simulink model "proj_ish"  (R2023a)
settings: Solver=FixedStepAuto  StartTime=0.0  StopTime=1000  FixedStep=0.01  RelTol=1e-3
values from neighbouring files (symbols this model uses):
  barrier_dist01 = 1300    [main_proj.m]
  barrier_dist02 = barrier_dist01+barrier_dist12    (= 10600)    [main_proj.m]
  barrier_dist03 = barrier_dist02+barrier_dist23    (= 21900)    [main_proj.m]
  barrier_dist04 = barrier_dist03+barrier_dist34    (= 53200)    [main_proj.m]
  L = 62832    [main_proj.m]
  start_times = [0 50 240]    [main_proj.m]
  train_acc_close = (30-50)/25    (= -0.8)    [main_proj.m]
  train_acc_passed = (50-30)/2.5    (= 8)    [main_proj.m]
  train_velocity_far = 50    [main_proj.m]
  trains = 3    [main_proj.m]
  V = 28    [main_proj.m]
  v = 0.15*V    (= 4.2)    [main_proj.m]
undefined symbols (not defined in the file or in its folder): a_cruise, a_cruise_stop, a_stop_start, converter_data, downtab, downth, emap, Iei, nevec, thvec, uptab, upth, vehicledata
(part 1 of 2)
settings Model: NumberOfSteps=100  Creator=Alex  LastModifiedBy=Alex

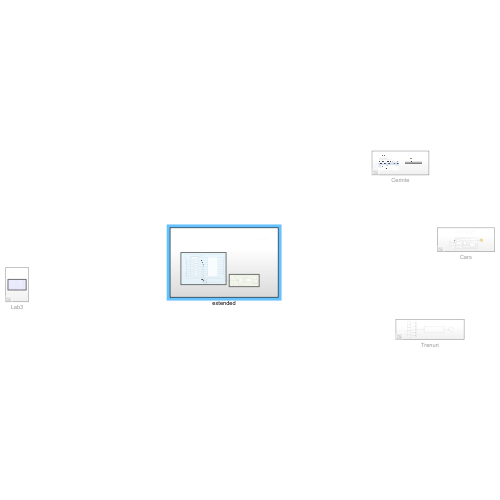
[thumbnail: Simulink's stored preview of the top-level diagram]
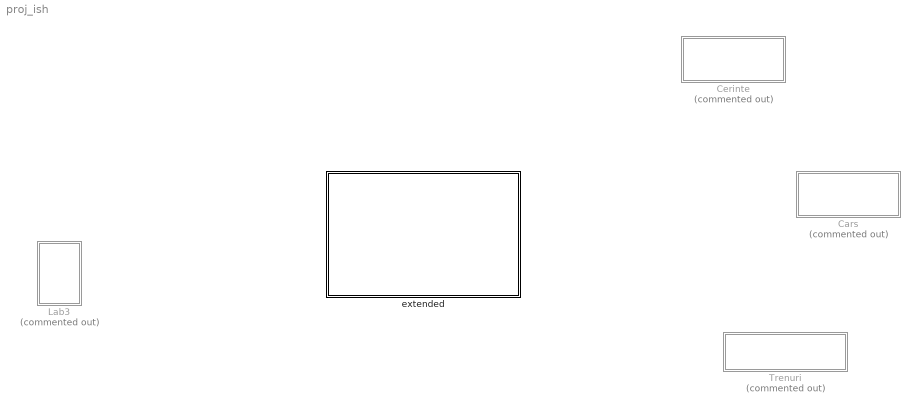
== system proj_ish ==
  Cars : Subsystem  Commented=on
  Cerinte : Subsystem  Commented=on
  Lab3 : Subsystem  Commented=on
  Trenuri : Subsystem  Commented=on
  extended : Subsystem

== system proj_ish/Cars ==
  Car : Subsystem  Commented=on
  Car Controller : Stateflow chart  Commented=on  TreatAsAtomicUnit=on
  Engine : Subsystem
  PlotResults : Scope  NumInputPorts=3
  Scope1 : Scope  Commented=on
  ShiftLogic : Stateflow chart  TreatAsAtomicUnit=on
  Step : Step  Time=50  Before=50  After=0  SampleTime=0
  Step1 : Step  Time=50  After=500  SampleTime=0
  Transmission : Subsystem
  Vehicle : Subsystem  mask(vehicle model){Rfd=vehicledata(1), rload0=vehicledata(2), rload2=vehicledata(3), Rw=vehicledata(4), Iv=vehicledata(5), N20=vehicledata(6)/vehicledata(4)*vehicledata(1)}
      mask prompts: Rfd "final drive ratio"; rload0 "drag friction at wheels"; rload2 "aerodynamic drag"; Rw "wheel radius"; Iv "vehicle inertia"; N20 "initial transmission output speed"
      mask help: vehicle dynamics: torque input from trans., outputs are input speed (transmission output) and vehicle speed
      mask Display: image('$imagefile') % use "Edit Image" on toolstrip to change.
  wires:
  Car/1(pozitie) -> Car Controller/1(pzoitie), Scope1/1
  Car Controller/1(stare_masina) -> Car/1(stare_masina)
  Transmission/2(Tout) -> Vehicle/1(OutputTorque)  "OutputTorque"
  Transmission/1(Ti) -> Engine/1(Ti)  "ImpellerTorque"
  ShiftLogic/1(Gear) -> Transmission/2(Gear)
  Engine/1(Ne) -> Transmission/1(Ne), PlotResults/2  "EngineRPM"
  Vehicle/1(VehicleSpeed) -> ShiftLogic/2(VehicleSpeed), PlotResults/3  "VehicleSpeed"
  Step1/1 -> Vehicle/2(BrakeTorque)  "Brake"
  Step/1 -> ShiftLogic/1(Throttle), Engine/2(Throttle), PlotResults/1  "Throttle"
  Vehicle/2(TransmissionRPM) -> Transmission/3(Nout)  "TransmissionRPM"

== system proj_ish/Cerinte ==
  note: trenul este in starea aproape, deci are viteza 30mps
      | evenimentul de "aproape" se genereaza la 1000m distanta de bariera
      | Durata propriu zisa de inchidere a barierei este 90/9=10 secunde
      | Trenul ajunge de la 1000m la 10m (pragul limita considerat) distanta de bariera in 990/30=33 secunde
      | Din cele 33 secunde, 10 se aloca pentru coborarea barierei
      | Deci intarzierea maxima pe care o poate avea controller-ul pentru a ne asigura ca bariera va fi complet inchisa la momentul in care trenul intra in intervalul +-10m este u=23 secunde
  note: r=10km => C=2*pi*r=62832m

== system proj_ish/Lab3 ==
  note: Lab 3
  Bariera : Subsystem  Commented=on
  Control bariera : Subsystem  Commented=on
  Controller : Stateflow chart  Commented=on  TreatAsAtomicUnit=on
  Scope : Scope  Commented=on  NumInputPorts=2
  Tren : Subsystem  Commented=on
  wires:
  Controller/1(starebariera) -> Bariera/1(stare_bariera)
  Bariera/1(y) -> Controller/1(y), Scope/2
  Controller/2(starectrl) -> Control bariera/1(stare_control)
  Control bariera/1(z) -> Controller/2(z)
  Tren/1(x) -> Controller/3(x), Scope/1
  Controller/3(staretren) -> Tren/1(stare_tren)

== system proj_ish/Trenuri ==
  Mux : Mux  Commented=on  Inputs=5
  Scope1 : Scope  Commented=on
  Step{,1..4} (5 alike) : Step  Commented=on  Time=0  SampleTime=0
  Trenuri : Subsystem  Commented=on
  wires:
  Step/1 -> Mux/1
  Mux/1 -> Trenuri/1(stari_trenuri)
  Step2/1 -> Mux/3
  Trenuri/1(x) -> Scope1/1
  Step3/1 -> Mux/4
  Step1/1 -> Mux/2
  Step4/1 -> Mux/5

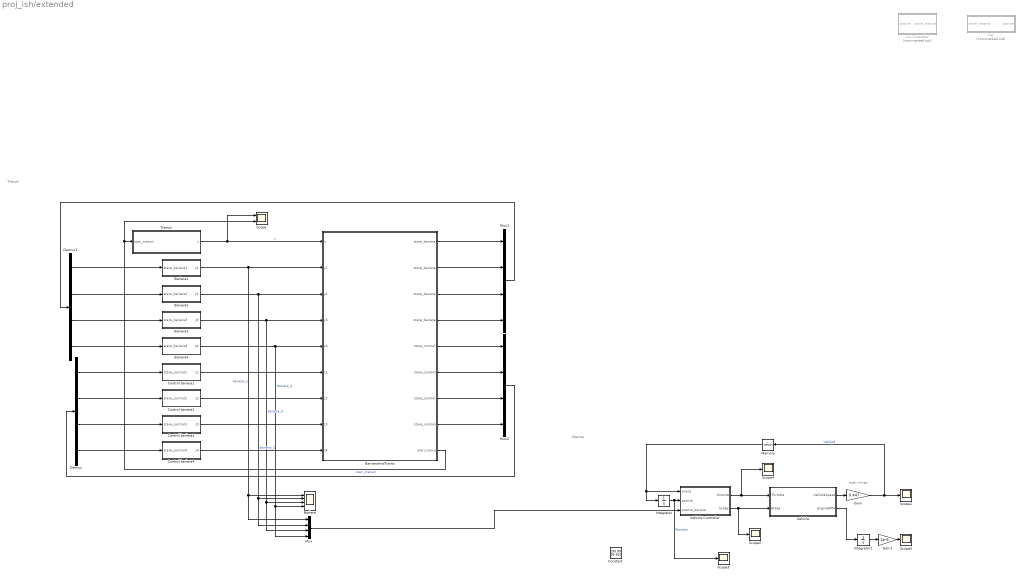
== system proj_ish/extended ==
  note: Masina
  note: Trenuri
  note: mph->mps
  Bariera1 : Subsystem
  Bariera2 : Subsystem
  Bariera3 : Subsystem
  Bariera4 : Subsystem
  Bariere : Scope  NumInputPorts=4
  BarriersAndTrains : Stateflow chart  TreatAsAtomicUnit=on
  Car : Subsystem  Commented=on
  Car Controller : Stateflow chart  Commented=on  TreatAsAtomicUnit=on
  Constant : Constant  Value=[90 90 90 90]
  Control bariera1 : Subsystem
  Control bariera2 : Subsystem
  Control bariera3 : Subsystem
  Control bariera4 : Subsystem
  Demux : Demux
  Demux1 : Demux
  Gain : Gain  Gain=0.447
  Gain1 : Gain  Gain=2e-6
  Integrator : Integrator
  Integrator1 : Integrator
  Memory : Memory
  Mux : Mux
  Mux1 : Mux
  Mux2 : Mux
  Scope : Scope  NumInputPorts=2
  Scope{1..5} (5 alike) : Scope
  Trenuri : Subsystem
  Vehicle : Subsystem
  Vehicle Controller : Stateflow chart  TreatAsAtomicUnit=on
      settings: PortSchema="{\"entries\":[{\"content\":{\"sides\":[{\"content\":{\"connectorIds\":[\"In2\",\"In1\",\"In3\"]},\"type\":\"ConnectorPlacement.EquallySpacedRectSide\",\"uuid\":\"df773432-b911-4b0c-bdef-38af23bc8129\"},{\"content\":{\"connectorIds\":[\"Out1\",\"Out2\"],\"side\":\"RIGHT\"},\"type\":\"ConnectorPlacement.EquallySpacedRectSide\",\"uuid\":\"5ca2d89f-a3cb-4395-9b83-e502d168ef7e\"},{\"content\":{\"side\":\"TOP\"},\"type\":\"ConnectorPlacement.EquallySpacedRectSide\",\"uuid\":\"7df5f796-226c-4e0d-a429-f20110d7350f\"}]},\"type\":\"ConnectorPlacement.EquallySpacedConnector\",\"uuid\":\"5b5bbf8d-caf4-492a-a09a-43efcf324f87\"}],\"packageUris\":[\"http://schema.mathworks.com/mf0/Connector/R2020b\"],\"version\":\"1.0\"}"
  wires:
  Trenuri/1(x) -> Scope/1, BarriersAndTrains/1(x)  "x"
  Bariera1/1(y1) -> Mux/1, Bariere/1, BarriersAndTrains/2(y1)  "bariera_1"
  Bariera2/1(y2) -> Mux/2, Bariere/2, BarriersAndTrains/3(y2)  "bariera_2"
  Bariera3/1(y3) -> Mux/3, Bariere/3, BarriersAndTrains/4(y3)  "bariera_3"
  Bariera4/1(y4) -> BarriersAndTrains/5(y4), Mux/4, Bariere/4  "bariera_4"
  Control bariera3/1(z3) -> BarriersAndTrains/8(z3)
  Control bariera2/1(z2) -> BarriersAndTrains/7(z2)
  Control bariera1/1(z1) -> BarriersAndTrains/6(z1)
  Control bariera4/1(z4) -> BarriersAndTrains/9(z4)
  BarriersAndTrains/2(stare_bariera2) -> Mux1/2
  BarriersAndTrains/1(stare_bariera1) -> Mux1/1
  BarriersAndTrains/3(stare_bariera3) -> Mux1/3
  BarriersAndTrains/4(stare_bariera4) -> Mux1/4
  BarriersAndTrains/5(stare_control1) -> Mux2/1
  BarriersAndTrains/6(stare_control2) -> Mux2/2
  BarriersAndTrains/7(stare_control3) -> Mux2/3
  BarriersAndTrains/8(stare_control4) -> Mux2/4
  Mux2/1 -> Demux/1
  Demux/3 -> Control bariera3/1(stare_control3)
  Demux/2 -> Control bariera2/1(stare_control2)
  Demux/4 -> Control bariera4/1(stare_control4)
  Demux/1 -> Control bariera1/1(stare_control1)
  Demux1/1 -> Bariera1/1(stare_bariera1)
  Demux1/2 -> Bariera2/1(stare_bariera2)
  Demux1/3 -> Bariera3/1(stare_bariera3)
  Demux1/4 -> Bariera4/1(stare_bariera4)
  Mux1/1 -> Demux1/1
  BarriersAndTrains/9(stari_trenuri) -> Scope/2, Trenuri/1(stari_trenuri)  "stari_trenuri"
  Vehicle Controller/2(brake) -> Scope2/1, Vehicle/2(Brake)
  Integrator/1 -> Scope3/1, Vehicle Controller/1(pozitie)  "Position"
  Gain/1 -> Memory/1, Scope1/1  "VehSpd"
  Vehicle Controller/1(throttle) -> Scope4/1, Vehicle/1(Throttle)
  Memory/1 -> Integrator/1, Vehicle Controller/2(viteza)
  Vehicle/1(VehicleSpeed) -> Gain/1
  Mux/1 -> Vehicle Controller/3(pozitie_bariere)
  Vehicle/2(EngineRPM) -> Integrator1/1
  Integrator1/1 -> Gain1/1
  Gain1/1 -> Scope5/1

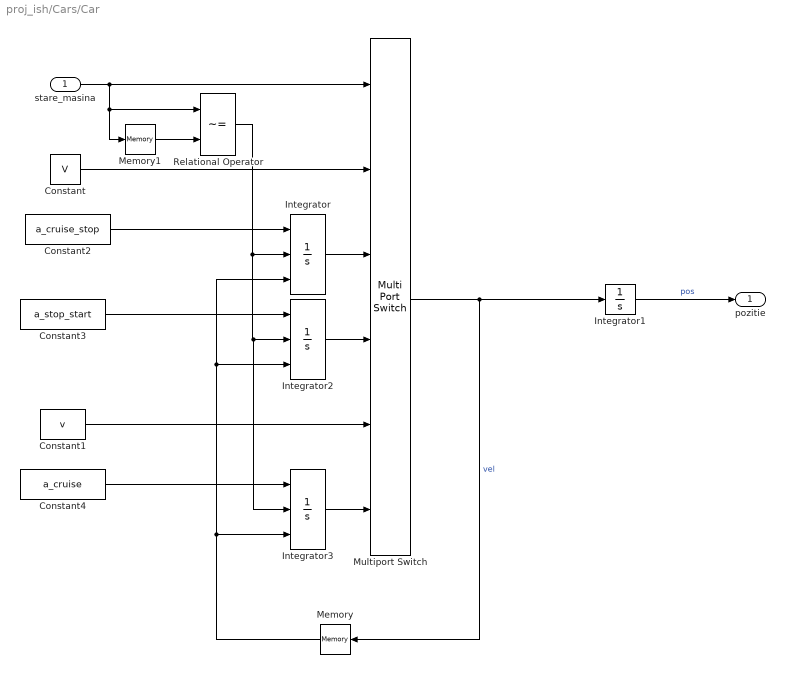
== system proj_ish/Cars/Car ==
  stare_masina : Inport
  Constant : Constant  Value=V
  Constant1 : Constant  Value=v
  Constant2 : Constant  Value=a_cruise_stop
  Constant3 : Constant  Value=a_stop_start
  Constant4 : Constant  Value=a_cruise
  Integrator : Integrator  ExternalReset=rising  InitialConditionSource=external  LimitOutput=on  UpperSaturationLimit=200  LowerSaturationLimit=0
  Integrator1 : Integrator
  Integrator2 : Integrator  ExternalReset=rising  InitialConditionSource=external  LimitOutput=on  UpperSaturationLimit=v  LowerSaturationLimit=0
  Integrator3 : Integrator  ExternalReset=rising  InitialConditionSource=external  LimitOutput=on  UpperSaturationLimit=V  LowerSaturationLimit=0
  Memory : Memory  InitialCondition=V
  Memory1 : Memory  InitialCondition=1
  Multiport Switch : MultiPortSwitch  Inputs=5  SaturateOnIntegerOverflow=off  InputSameDT=off
  Relational Operator : RelationalOperator  Operator=~=  OutDataTypeStr=boolean  RndMeth=Simplest  InputSameDT=off
  pozitie : Outport
  wires:
  Multiport Switch/1 -> Memory/1, Integrator1/1  "vel"
  stare_masina/1 -> Multiport Switch/1, Memory1/1, Relational Operator/1
  Integrator1/1 -> pozitie/1  "pos"
  Constant/1 -> Multiport Switch/2
  Integrator/1 -> Multiport Switch/3
  Integrator2/1 -> Multiport Switch/4
  Constant1/1 -> Multiport Switch/5
  Integrator3/1 -> Multiport Switch/6
  Memory/1 -> Integrator3/3, Integrator2/3, Integrator/3
  Memory1/1 -> Relational Operator/2
  Relational Operator/1 -> Integrator3/2, Integrator2/2, Integrator/2
  Constant2/1 -> Integrator/1
  Constant3/1 -> Integrator2/1
  Constant4/1 -> Integrator3/1

== system proj_ish/Cars/Engine ==
  note: Engine
  Ti : Inport  Unit=ft*lbf@torque
  Throttle : Inport  Port=2  Unit=%
  EnginePlusImpellerInertia : Gain  Gain=1/Iei  SaturateOnIntegerOverflow=on  OutDataTypeStr=Inherit: Same as input  ParamDataTypeStr=Inherit: Same as input
  EngineTorque : Lookup_n-D  BreakpointsForDimension1=thvec  BreakpointsForDimension2=nevec  Table=emap
      settings: InputPortMap=u0,u1
  Integrator : Integrator  InitialCondition=1000  LimitOutput=on  UpperSaturationLimit=6000  LowerSaturationLimit=600  ZeroCross=off
  Sum : Sum  Inputs=-+  InputSameDT=on  SaturateOnIntegerOverflow=on  OutDataTypeStr=Inherit: Same as first input
  Ne : Outport  Unit=rpm  VectorParamsAs1DForOutWhenUnconnected=off
  wires:
  Ti/1 -> Sum/1
  Throttle/1 -> EngineTorque/1
  Integrator/1 -> EngineTorque/2, Ne/1
  Sum/1 -> EnginePlusImpellerInertia/1
  EnginePlusImpellerInertia/1 -> Integrator/1
  EngineTorque/1 -> Sum/2

== system proj_ish/Cars/ShiftLogic/ComputeThreshold ==
  note: Threshold Calculation
  Gear : Inport
  Throttle : Inport  Port=2
  f : TriggerPort  TriggerType=function-call  VariantControl=(inherit)
      settings: CopyFcn=Stateflow.SLINSF.SimulinkMan.removeBlockPreDeleteFcn  PreDeleteFcn=Stateflow.SLINSF.SimulinkMan.unsafePredeleteFcn
  InterpDown : Lookup_n-D  BreakpointsForDimension1=downth  BreakpointsForDimension2=[1:4]  Table=downtab  OutDataTypeStr=double  InputSameDT=off  LockScale=on
      settings: InputPortMap=u0,u1
  InterpUp : Lookup_n-D  BreakpointsForDimension1=upth  BreakpointsForDimension2=[1:4]  Table=uptab  OutDataTypeStr=double  InputSameDT=off  LockScale=on
      settings: InputPortMap=u0,u1
  down_th : Outport  InitialOutput=0  VectorParamsAs1DForOutWhenUnconnected=off
  up_th : Outport  Port=2  InitialOutput=0  VectorParamsAs1DForOutWhenUnconnected=off
  wires:
  InterpUp/1 -> up_th/1
  InterpDown/1 -> down_th/1
  Throttle/1 -> InterpDown/1, InterpUp/1
  Gear/1 -> InterpDown/2, InterpUp/2

== system proj_ish/Cars/Transmission ==
  note: Transmission
  Ne : Inport  Unit=rpm
  Gear : Inport  Port=2  Unit=1
  Nout : Inport  Port=3  Unit=rpm
  TorqueConverter : Subsystem  mask(torque converter){speedratio=converter_data(:,1), Kfactor=converter_data(:,2), Torkratio=converter_data(:,3)}
      mask prompts: speedratio "speed ratio"; Kfactor "K factor"; Torkratio "torque ratio"
      mask help: torque converter
      mask Help: Torque converter input and output torques are computed as a function of the input and output speeds
      mask Display: plot([cos([90:10:450]*pi/180),.63*cos([90:10:450]*pi/180),.63*cos([90:10:240]*pi/180),cos([240:10:300]*pi/180),.63*cos([300]*pi/180)],[sin([90:10:450]*pi/180),.63*sin([90:10:450]*pi/180)+.1,.63*sin([90:10:240]*pi/180)+.1,sin([240:10:300]*pi/180),.63*sin([300]*pi/180)+.1])
  TransmissionRatio : Subsystem
  Ti : Outport  Unit=ft*lbf@torque  VectorParamsAs1DForOutWhenUnconnected=off
  Tout : Outport  Port=2  Unit=ft*lbf@torque  VectorParamsAs1DForOutWhenUnconnected=off
  wires:
  TransmissionRatio/1(Tout) -> Tout/1
  TorqueConverter/1(Ti) -> Ti/1
  Nout/1 -> TransmissionRatio/3(Nout)
  Gear/1 -> TransmissionRatio/2(Gear)
  Ne/1 -> TorqueConverter/1(Ne)
  TransmissionRatio/2(Nin) -> TorqueConverter/2(Nin)
  TorqueConverter/2(Tt) -> TransmissionRatio/1(Tin)  "TurbineTorque"

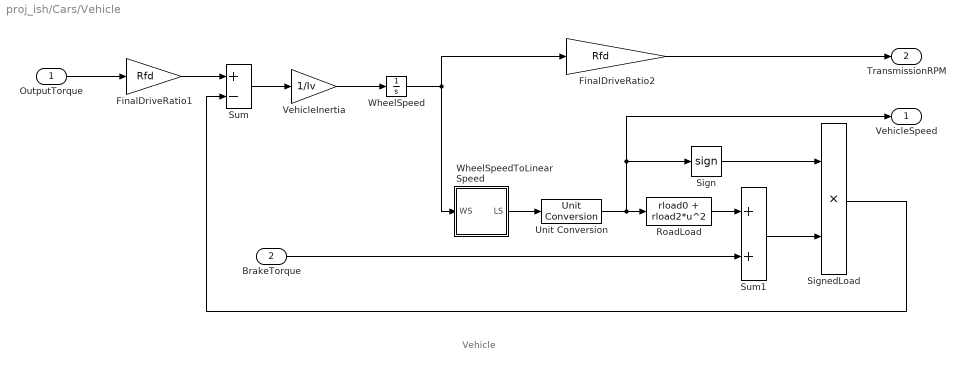
== system proj_ish/Cars/Vehicle ==
  note: Vehicle
  OutputTorque : Inport  Unit=ft*lbf@torque
  BrakeTorque : Inport  Port=2  Unit=ft*lbf@torque
  FinalDriveRatio1 : Gain  Gain=Rfd  SaturateOnIntegerOverflow=on  OutDataTypeStr=Inherit: Same as input  ParamDataTypeStr=Inherit: Same as input
  FinalDriveRatio2 : Gain  Gain=Rfd  SaturateOnIntegerOverflow=on  OutDataTypeStr=Inherit: Same as input  ParamDataTypeStr=Inherit: Same as input
  RoadLoad : Fcn  Expr=rload0 + rload2*u^2
  Sign : Signum
  SignedLoad : Product  InputSameDT=on  SaturateOnIntegerOverflow=on  OutDataTypeStr=Inherit: Same as first input
  Sum : Sum  Inputs=+-  InputSameDT=on  SaturateOnIntegerOverflow=on  OutDataTypeStr=Inherit: Same as first input
  Sum1 : Sum  InputSameDT=on  SaturateOnIntegerOverflow=on  OutDataTypeStr=Inherit: Same as first input
  Unit Conversion : UnitConversion
  VehicleInertia : Gain  Gain=1/Iv  SaturateOnIntegerOverflow=on  OutDataTypeStr=Inherit: Same as input  ParamDataTypeStr=Inherit: Same as input
  WheelSpeed : Integrator  InitialCondition=N20/Rfd  ZeroCross=off
  WheelSpeedToLinearSpeed : Subsystem
  VehicleSpeed : Outport  Unit=mph  VectorParamsAs1DForOutWhenUnconnected=off
  TransmissionRPM : Outport  Port=2  Unit=rpm  VectorParamsAs1DForOutWhenUnconnected=off
  wires:
  FinalDriveRatio2/1 -> TransmissionRPM/1
  BrakeTorque/1 -> Sum1/2
  Sum1/1 -> SignedLoad/2
  RoadLoad/1 -> Sum1/1
  Sign/1 -> SignedLoad/1
  SignedLoad/1 -> Sum/2
  OutputTorque/1 -> FinalDriveRatio1/1
  VehicleInertia/1 -> WheelSpeed/1
  Sum/1 -> VehicleInertia/1
  Unit Conversion/1 -> VehicleSpeed/1, Sign/1, RoadLoad/1
  WheelSpeed/1 -> WheelSpeedToLinearSpeed/1(WS), FinalDriveRatio2/1
  FinalDriveRatio1/1 -> Sum/1
  WheelSpeedToLinearSpeed/1(LS) -> Unit Conversion/1

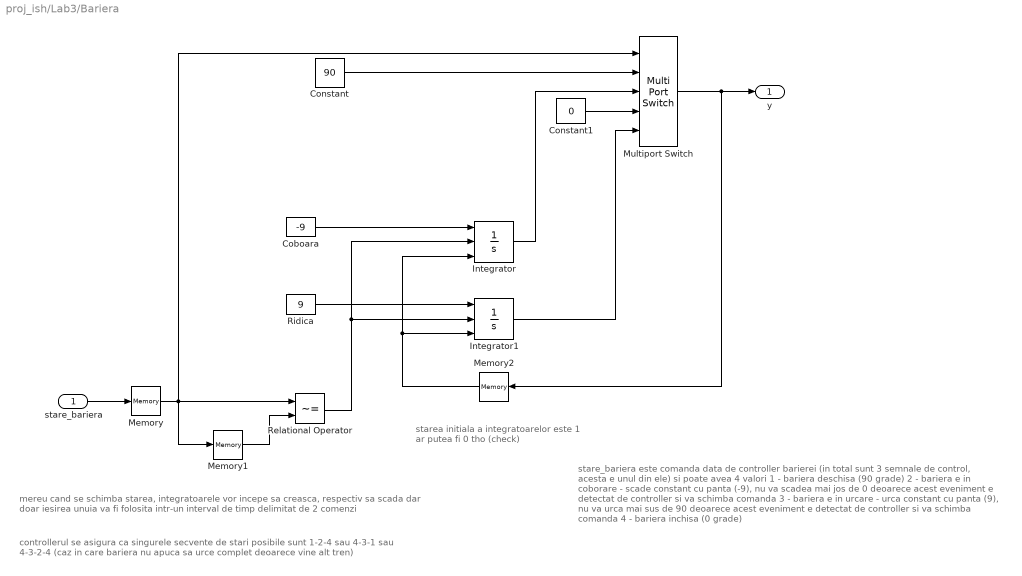
== system proj_ish/Lab3/Bariera ==
  note: controllerul se asigura ca singurele secvente de stari posibile sunt
      | 1-2-4
      | sau
      | 4-3-1
      | sau 4-3-2-4 (caz in care bariera nu apuca sa urce complet deoarece vine alt tren)
  note: mereu cand se schimba starea, integratoarele vor incepe sa creasca, respectiv sa scada
      | dar doar iesirea unuia va fi folosita intr-un interval de timp delimitat de 2 comenzi
  note: starea initiala a integratoarelor este 1
      | ar putea fi 0 tho (check)
  note: stare_bariera este comanda data de controller barierei (in total sunt 3 semnale de control, acesta e unul din ele) si poate avea 4 valori
      | 1 - bariera deschisa (90 grade)
      | 2 - bariera e in coborare - scade constant cu panta (-9), nu va scadea mai jos de 0 deoarece acest eveniment e detectat de controller si va schimba comanda
      | 3 - bariera e in urcare - urca constant cu panta (9), nu va urca mai sus de 90 deoarece acest eveniment e detectat de controller si va schimba comanda
      | 4 - bariera inchisa (0 grade)
  stare_bariera : Inport
  Coboara : Constant  Value=-9
  Constant : Constant  Value=90
  Constant1 : Constant  Value=0
  Integrator : Integrator  ExternalReset=rising  InitialConditionSource=external
  Integrator1 : Integrator  ExternalReset=rising  InitialConditionSource=external
  Memory : Memory  InitialCondition=1
  Memory1 : Memory  InitialCondition=1
  Memory2 : Memory
  Multiport Switch : MultiPortSwitch  Inputs=4  SaturateOnIntegerOverflow=off  InputSameDT=off
  Relational Operator : RelationalOperator  Operator=~=  OutDataTypeStr=boolean  RndMeth=Simplest  InputSameDT=off
  Ridica : Constant  Value=9
  y : Outport
  wires:
  Multiport Switch/1 -> Memory2/1, y/1
  Constant/1 -> Multiport Switch/2
  Coboara/1 -> Integrator/1
  Ridica/1 -> Integrator1/1
  Integrator/1 -> Multiport Switch/3
  stare_bariera/1 -> Memory/1
  Memory/1 -> Multiport Switch/1, Memory1/1, Relational Operator/1
  Memory1/1 -> Relational Operator/2
  Relational Operator/1 -> Integrator1/2, Integrator/2
  Integrator1/1 -> Multiport Switch/5
  Constant1/1 -> Multiport Switch/4
  Memory2/1 -> Integrator/3, Integrator1/3

== system proj_ish/Lab3/Control bariera ==
  note: iesirea z masoara cat timp a trecut de la ultima comanda de tip ridicare sau coborare
      | (scopul este modelarea unui delay intre momentul in care se ia decizia si momentul in care bariera executa comanda, modelarea propriu zisa se face in controller)
      |
      | daca controllerul e in starea de asteptare, atunci z=0
      | daca controllerul hotaraste comanda de ridicare sau coborare, se porneste un timer care se opreste cand are loc una din tranzitiile {3->1} {2->1} {3->2}
  note: stare_control este starea decizionala in care se afla controllerul
      | 1 - asteptare
      | 2 - comanda coborare
      | 3 - comanda ridicare
  stare_control : Inport
  Constant : Constant  Value=0
  Constant1 : Constant
  Constant2 : Constant
  Integrator : Integrator  ExternalReset=rising
  Memory : Memory  InitialCondition=1
  Memory1 : Memory  InitialCondition=1
  Multiport Switch : MultiPortSwitch  DataPortOrder=Specify indices  Inputs=2  DataPortIndices={0,1}  SaturateOnIntegerOverflow=off  InputSameDT=off
  Relational Operator : RelationalOperator  Operator=~=  OutDataTypeStr=boolean  RndMeth=Simplest  InputSameDT=off
  Relational Operator1 : RelationalOperator  Operator===  OutDataTypeStr=boolean  RndMeth=Simplest  InputSameDT=off
  z : Outport
  wires:
  Multiport Switch/1 -> z/1
  Constant/1 -> Multiport Switch/3
  stare_control/1 -> Relational Operator/1, Memory/1
  Memory/1 -> Relational Operator/2, Relational Operator1/1
  Constant1/1 -> Integrator/1
  Relational Operator/1 -> Integrator/2
  Integrator/1 -> Memory1/1
  Memory1/1 -> Multiport Switch/2
  Constant2/1 -> Relational Operator1/2
  Relational Operator1/1 -> Multiport Switch/1

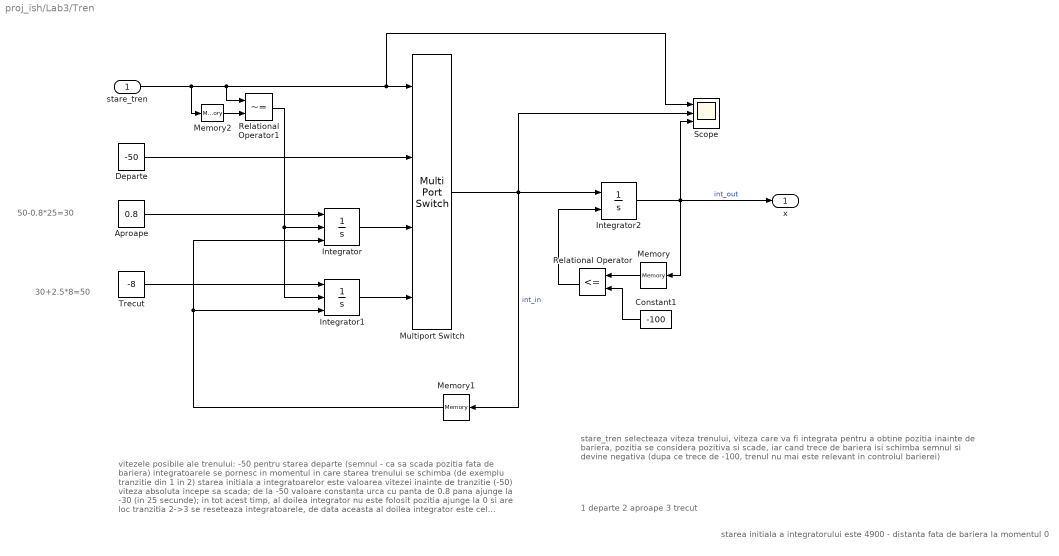
== system proj_ish/Lab3/Tren ==
  note: 30+2.5*8=50
  note: starea initiala a integratorului este 4900 - distanta fata de bariera la momentul 0
  note: 1 departe
      | 2 aproape
      | 3 trecut
  note: vitezele posibile ale trenului:
      | -50 pentru starea departe (semnul - ca sa scada pozitia fata de bariera)
      |
      | integratoarele se pornesc in momentul in care starea trenului se schimba (de exemplu tranzitie din 1 in 2)
      |
      | starea initiala a integratoarelor este valoarea vitezei inainte de tranzitie (-50)
      | viteza absoluta incepe sa scada; de la -50 valoare constanta urca cu panta de 0.8 pana ajunge la -30 (in 25 secunde); in tot acest timp, al doilea integrator nu este folosit
      |
      | pozitia ajunge la 0 si are loc tranzitia 2->3
      |
      | se reseteaza integratoarele, de data aceasta al doilea integrator este cel folosit; el are starea initiala -30 si scade cu o panta de -8
  note: 50-0.8*25=30
  note: stare_tren selecteaza viteza trenului, viteza care va fi integrata pentru a obtine pozitia
      | inainte de bariera, pozitia se considera pozitiva si scade, iar cand trece de bariera isi schimba semnul si devine negativa (dupa ce trece de -100, trenul nu mai este relevant in controlul barierei)
  stare_tren : Inport
  Aproape : Constant  Value=0.8
  Constant1 : Constant  Value=-100
  Departe : Constant  Value=-50
  Integrator : Integrator  ExternalReset=rising  InitialConditionSource=external
  Integrator1 : Integrator  ExternalReset=rising  InitialConditionSource=external
  Integrator2 : Integrator  ExternalReset=rising  InitialCondition=4900
  Memory : Memory
  Memory1 : Memory
  Memory2 : Memory  InitialCondition=1
  Multiport Switch : MultiPortSwitch  SaturateOnIntegerOverflow=off  InputSameDT=off
  Relational Operator : RelationalOperator  Operator=<=  OutDataTypeStr=boolean  RndMeth=Simplest  InputSameDT=off
  Relational Operator1 : RelationalOperator  Operator=~=  OutDataTypeStr=boolean  RndMeth=Simplest  InputSameDT=off
  Scope : Scope  NumInputPorts=3
  Trecut : Constant  Value=-8
  x : Outport
  wires:
  Departe/1 -> Multiport Switch/2
  stare_tren/1 -> Memory2/1, Scope/1, Multiport Switch/1, Relational Operator1/1
  Aproape/1 -> Integrator/1
  Trecut/1 -> Integrator1/1
  Integrator2/1 -> Scope/3, x/1, Memory/1  "int_out"
  Constant1/1 -> Relational Operator/2
  Memory/1 -> Relational Operator/1
  Relational Operator/1 -> Integrator2/2
  Multiport Switch/1 -> Scope/2, Memory1/1, Integrator2/1  "int_in"
  Integrator/1 -> Multiport Switch/3
  Integrator1/1 -> Multiport Switch/4
  Memory1/1 -> Integrator/3, Integrator1/3
  Memory2/1 -> Relational Operator1/2
  Relational Operator1/1 -> Integrator/2, Integrator1/2

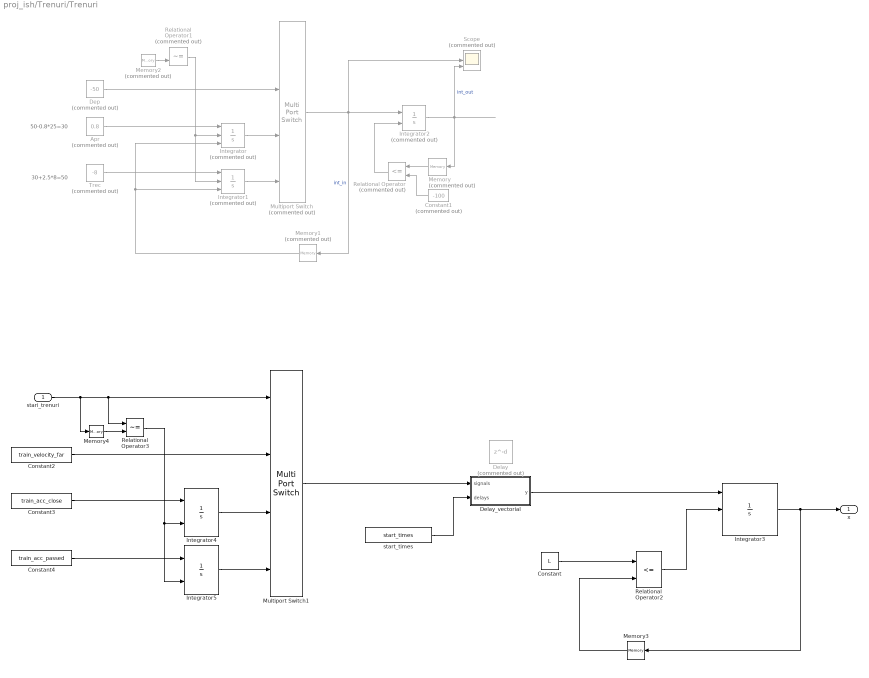
== system proj_ish/Trenuri/Trenuri ==
  note: 30+2.5*8=50
  note: 50-0.8*25=30
  stari_trenuri : Inport
  Apr : Constant  Commented=on  Value=0.8
  Constant : Constant  Value=L
  Constant1 : Constant  Commented=on  Value=-100
  Constant2 : Constant  Value=train_velocity_far
  Constant3 : Constant  Value=train_acc_close
  Constant4 : Constant  Value=train_acc_passed
  Delay : Delay  Commented=on  DelayLengthSource=Input port
      settings: InputPortMap=u0,p1
  Delay_vectorial : MATLAB Function  TreatAsAtomicUnit=on
  Dep : Constant  Commented=on  Value=-50
  Integrator : Integrator  Commented=on  ExternalReset=rising  InitialConditionSource=external
  Integrator1 : Integrator  Commented=on  ExternalReset=rising  InitialConditionSource=external
  Integrator2 : Integrator  Commented=on  ExternalReset=rising  InitialCondition=4900
  Integrator3 : Integrator  ExternalReset=rising  InitialConditionSource=external
  Integrator4 : Integrator  ExternalReset=rising
  Integrator5 : Integrator  ExternalReset=rising
  Memory : Memory  Commented=on
  Memory1 : Memory  Commented=on
  Memory2 : Memory  Commented=on  InitialCondition=1
  Memory3 : Memory
  Memory4 : Memory  InitialCondition=ones(1,trains)
  Multiport Switch : MultiPortSwitch  Commented=on  SaturateOnIntegerOverflow=off  InputSameDT=off
  Multiport Switch1 : MultiPortSwitch  SaturateOnIntegerOverflow=off  InputSameDT=off
  Relational Operator : RelationalOperator  Commented=on  Operator=<=  OutDataTypeStr=boolean  RndMeth=Simplest  InputSameDT=off
  Relational Operator1 : RelationalOperator  Commented=on  Operator=~=  OutDataTypeStr=boolean  RndMeth=Simplest  InputSameDT=off
  Relational Operator2 : RelationalOperator  Operator=<=  OutDataTypeStr=boolean  RndMeth=Simplest  InputSameDT=off
  Relational Operator3 : RelationalOperator  Operator=~=  OutDataTypeStr=boolean  RndMeth=Simplest  InputSameDT=off
  Scope : Scope  Commented=on  NumInputPorts=3
  Trec : Constant  Commented=on  Value=-8
  start_times : Constant  Value=start_times
  x : Outport
  wires:
  Dep/1 -> Multiport Switch/2
  ? -> Memory2/1, Scope/1, Multiport Switch/1, Relational Operator1/1
  Apr/1 -> Integrator/1
  Trec/1 -> Integrator1/1
  Integrator2/1 -> Scope/3, Memory/1  "int_out"
  Constant1/1 -> Relational Operator/2
  Memory/1 -> Relational Operator/1
  Relational Operator/1 -> Integrator2/2
  Multiport Switch/1 -> Scope/2, Memory1/1, Integrator2/1  "int_in"
  Integrator/1 -> Multiport Switch/3
  Integrator1/1 -> Multiport Switch/4
  Memory1/1 -> Integrator/3, Integrator1/3
  Memory2/1 -> Relational Operator1/2
  Relational Operator1/1 -> Integrator/2, Integrator1/2
  Multiport Switch1/1 -> Delay_vectorial/1(signals)
  stari_trenuri/1 -> Multiport Switch1/1, Relational Operator3/1, Memory4/1
  Integrator3/1 -> Memory3/1, x/1
  Constant2/1 -> Multiport Switch1/2
  start_times/1 -> Delay_vectorial/2(delays)
  Integrator4/1 -> Multiport Switch1/3
  Integrator5/1 -> Multiport Switch1/4
  Delay_vectorial/1(y) -> Integrator3/1
  Memory3/1 -> Relational Operator2/2
  Constant/1 -> Relational Operator2/1
  Relational Operator2/1 -> Integrator3/2
  Constant3/1 -> Integrator4/1
  Constant4/1 -> Integrator5/1
  Memory4/1 -> Relational Operator3/2
  Relational Operator3/1 -> Integrator4/2, Integrator5/2

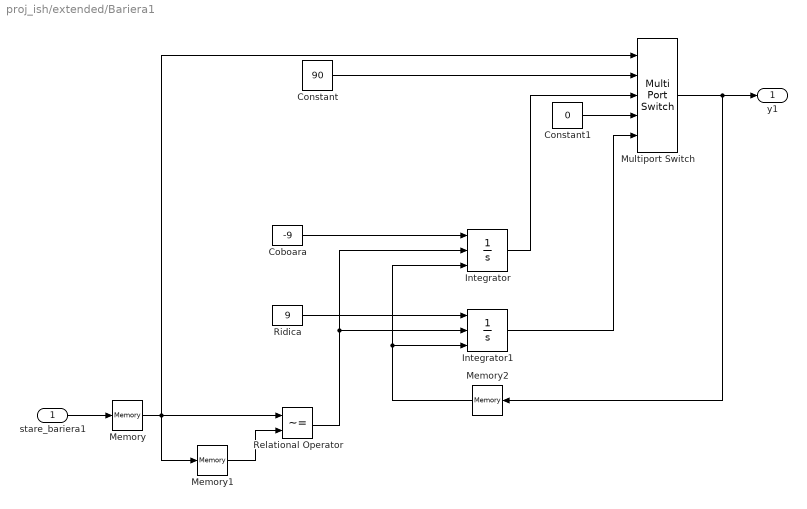
== system proj_ish/extended/Bariera1 ==
  stare_bariera1 : Inport
  Coboara : Constant  Value=-9
  Constant : Constant  Value=90
  Constant1 : Constant  Value=0
  Integrator : Integrator  ExternalReset=rising  InitialConditionSource=external
  Integrator1 : Integrator  ExternalReset=rising  InitialConditionSource=external
  Memory : Memory  InitialCondition=1
  Memory1 : Memory  InitialCondition=1
  Memory2 : Memory
  Multiport Switch : MultiPortSwitch  Inputs=4  SaturateOnIntegerOverflow=off  InputSameDT=off
  Relational Operator : RelationalOperator  Operator=~=  OutDataTypeStr=boolean  RndMeth=Simplest  InputSameDT=off
  Ridica : Constant  Value=9
  y1 : Outport
  wires:
  Multiport Switch/1 -> Memory2/1, y1/1
  Constant/1 -> Multiport Switch/2
  Coboara/1 -> Integrator/1
  Ridica/1 -> Integrator1/1
  Integrator/1 -> Multiport Switch/3
  stare_bariera1/1 -> Memory/1
  Memory/1 -> Multiport Switch/1, Memory1/1, Relational Operator/1
  Memory1/1 -> Relational Operator/2
  Relational Operator/1 -> Integrator1/2, Integrator/2
  Integrator1/1 -> Multiport Switch/5
  Constant1/1 -> Multiport Switch/4
  Memory2/1 -> Integrator/3, Integrator1/3

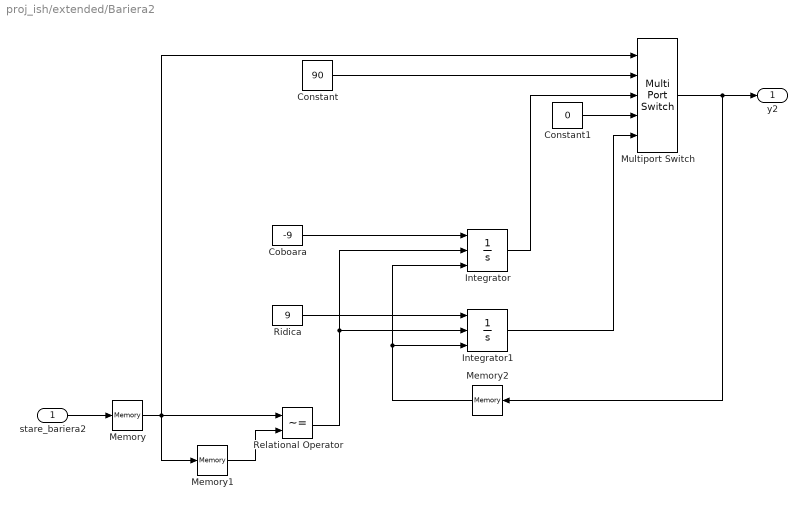
== system proj_ish/extended/Bariera2 ==
  stare_bariera2 : Inport
  Coboara : Constant  Value=-9
  Constant : Constant  Value=90
  Constant1 : Constant  Value=0
  Integrator : Integrator  ExternalReset=rising  InitialConditionSource=external
  Integrator1 : Integrator  ExternalReset=rising  InitialConditionSource=external
  Memory : Memory  InitialCondition=1
  Memory1 : Memory  InitialCondition=1
  Memory2 : Memory
  Multiport Switch : MultiPortSwitch  Inputs=4  SaturateOnIntegerOverflow=off  InputSameDT=off
  Relational Operator : RelationalOperator  Operator=~=  OutDataTypeStr=boolean  RndMeth=Simplest  InputSameDT=off
  Ridica : Constant  Value=9
  y2 : Outport
  wires:
  Memory2/1 -> Integrator1/3, Integrator/3
  Constant1/1 -> Multiport Switch/4
  Integrator1/1 -> Multiport Switch/5
  Relational Operator/1 -> Integrator/2, Integrator1/2
  Memory1/1 -> Relational Operator/2
  Memory/1 -> Relational Operator/1, Memory1/1, Multiport Switch/1
  stare_bariera2/1 -> Memory/1
  Integrator/1 -> Multiport Switch/3
  Ridica/1 -> Integrator1/1
  Coboara/1 -> Integrator/1
  Constant/1 -> Multiport Switch/2
  Multiport Switch/1 -> y2/1, Memory2/1

== system proj_ish/extended/Bariera3 ==
  stare_bariera3 : Inport
  Coboara : Constant  Value=-9
  Constant : Constant  Value=90
  Constant1 : Constant  Value=0
  Integrator : Integrator  ExternalReset=rising  InitialConditionSource=external
  Integrator1 : Integrator  ExternalReset=rising  InitialConditionSource=external
  Memory : Memory  InitialCondition=1
  Memory1 : Memory  InitialCondition=1
  Memory2 : Memory
  Multiport Switch : MultiPortSwitch  Inputs=4  SaturateOnIntegerOverflow=off  InputSameDT=off
  Relational Operator : RelationalOperator  Operator=~=  OutDataTypeStr=boolean  RndMeth=Simplest  InputSameDT=off
  Ridica : Constant  Value=9
  y3 : Outport
  wires:
  Multiport Switch/1 -> Memory2/1, y3/1
  Constant/1 -> Multiport Switch/2
  Coboara/1 -> Integrator/1
  Ridica/1 -> Integrator1/1
  Integrator/1 -> Multiport Switch/3
  stare_bariera3/1 -> Memory/1
  Memory/1 -> Multiport Switch/1, Memory1/1, Relational Operator/1
  Memory1/1 -> Relational Operator/2
  Relational Operator/1 -> Integrator1/2, Integrator/2
  Integrator1/1 -> Multiport Switch/5
  Constant1/1 -> Multiport Switch/4
  Memory2/1 -> Integrator/3, Integrator1/3

== system proj_ish/extended/Bariera4 ==
  stare_bariera4 : Inport
  Coboara : Constant  Value=-9
  Constant : Constant  Value=90
  Constant1 : Constant  Value=0
  Integrator : Integrator  ExternalReset=rising  InitialConditionSource=external
  Integrator1 : Integrator  ExternalReset=rising  InitialConditionSource=external
  Memory : Memory  InitialCondition=1
  Memory1 : Memory  InitialCondition=1
  Memory2 : Memory
  Multiport Switch : MultiPortSwitch  Inputs=4  SaturateOnIntegerOverflow=off  InputSameDT=off
  Relational Operator : RelationalOperator  Operator=~=  OutDataTypeStr=boolean  RndMeth=Simplest  InputSameDT=off
  Ridica : Constant  Value=9
  y4 : Outport
  wires:
  Memory2/1 -> Integrator1/3, Integrator/3
  Constant1/1 -> Multiport Switch/4
  Integrator1/1 -> Multiport Switch/5
  Relational Operator/1 -> Integrator/2, Integrator1/2
  Memory1/1 -> Relational Operator/2
  Memory/1 -> Relational Operator/1, Memory1/1, Multiport Switch/1
  stare_bariera4/1 -> Memory/1
  Integrator/1 -> Multiport Switch/3
  Ridica/1 -> Integrator1/1
  Coboara/1 -> Integrator/1
  Constant/1 -> Multiport Switch/2
  Multiport Switch/1 -> y4/1, Memory2/1

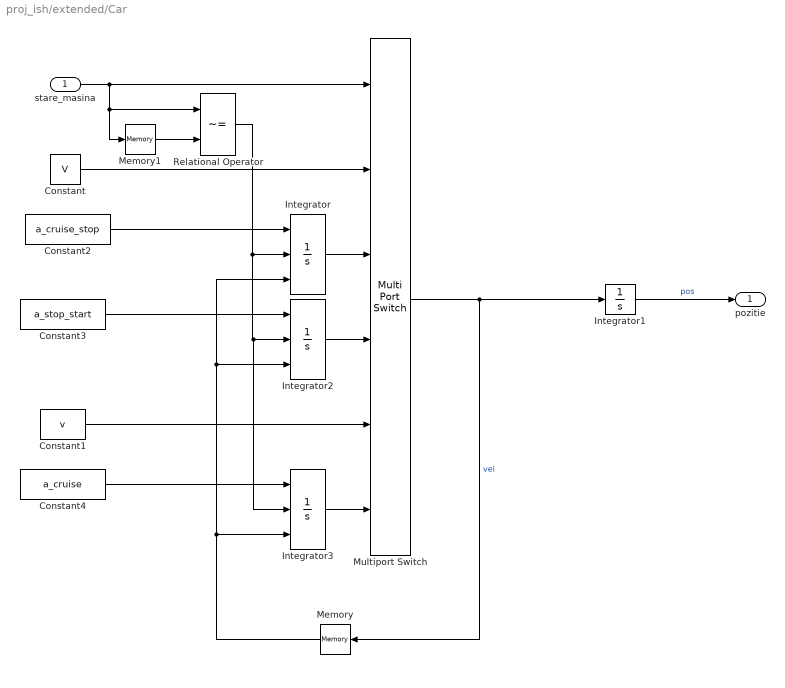
== system proj_ish/extended/Car ==
  stare_masina : Inport
  Constant : Constant  Value=V
  Constant1 : Constant  Value=v
  Constant2 : Constant  Value=a_cruise_stop
  Constant3 : Constant  Value=a_stop_start
  Constant4 : Constant  Value=a_cruise
  Integrator : Integrator  ExternalReset=rising  InitialConditionSource=external  LimitOutput=on  UpperSaturationLimit=200  LowerSaturationLimit=0
  Integrator1 : Integrator
  Integrator2 : Integrator  ExternalReset=rising  InitialConditionSource=external  LimitOutput=on  UpperSaturationLimit=v  LowerSaturationLimit=0
  Integrator3 : Integrator  ExternalReset=rising  InitialConditionSource=external  LimitOutput=on  UpperSaturationLimit=V  LowerSaturationLimit=0
  Memory : Memory  InitialCondition=V
  Memory1 : Memory  InitialCondition=1
  Multiport Switch : MultiPortSwitch  Inputs=5  SaturateOnIntegerOverflow=off  InputSameDT=off
  Relational Operator : RelationalOperator  Operator=~=  OutDataTypeStr=boolean  RndMeth=Simplest  InputSameDT=off
  pozitie : Outport
  wires:
  Multiport Switch/1 -> Memory/1, Integrator1/1  "vel"
  stare_masina/1 -> Multiport Switch/1, Memory1/1, Relational Operator/1
  Integrator1/1 -> pozitie/1  "pos"
  Constant/1 -> Multiport Switch/2
  Integrator/1 -> Multiport Switch/3
  Integrator2/1 -> Multiport Switch/4
  Constant1/1 -> Multiport Switch/5
  Integrator3/1 -> Multiport Switch/6
  Memory/1 -> Integrator3/3, Integrator2/3, Integrator/3
  Memory1/1 -> Relational Operator/2
  Relational Operator/1 -> Integrator3/2, Integrator2/2, Integrator/2
  Constant2/1 -> Integrator/1
  Constant3/1 -> Integrator2/1
  Constant4/1 -> Integrator3/1

== system proj_ish/extended/Control bariera1 ==
  stare_control1 : Inport
  Constant : Constant  Value=0
  Constant1 : Constant
  Constant2 : Constant
  Integrator : Integrator  ExternalReset=rising
  Memory : Memory  InitialCondition=1
  Memory1 : Memory  InitialCondition=1
  Multiport Switch : MultiPortSwitch  DataPortOrder=Specify indices  Inputs=2  DataPortIndices={0,1}  SaturateOnIntegerOverflow=off  InputSameDT=off
  Relational Operator : RelationalOperator  Operator=~=  OutDataTypeStr=boolean  RndMeth=Simplest  InputSameDT=off
  Relational Operator1 : RelationalOperator  Operator===  OutDataTypeStr=boolean  RndMeth=Simplest  InputSameDT=off
  z1 : Outport
  wires:
  Multiport Switch/1 -> z1/1
  Constant/1 -> Multiport Switch/3
  stare_control1/1 -> Relational Operator/1, Memory/1
  Memory/1 -> Relational Operator/2, Relational Operator1/1
  Constant1/1 -> Integrator/1
  Relational Operator/1 -> Integrator/2
  Integrator/1 -> Memory1/1
  Memory1/1 -> Multiport Switch/2
  Constant2/1 -> Relational Operator1/2
  Relational Operator1/1 -> Multiport Switch/1

== system proj_ish/extended/Control bariera2 ==
  stare_control2 : Inport
  Constant : Constant  Value=0
  Constant1 : Constant
  Constant2 : Constant
  Integrator : Integrator  ExternalReset=rising
  Memory : Memory  InitialCondition=1
  Memory1 : Memory  InitialCondition=1
  Multiport Switch : MultiPortSwitch  DataPortOrder=Specify indices  Inputs=2  DataPortIndices={0,1}  SaturateOnIntegerOverflow=off  InputSameDT=off
  Relational Operator : RelationalOperator  Operator=~=  OutDataTypeStr=boolean  RndMeth=Simplest  InputSameDT=off
  Relational Operator1 : RelationalOperator  Operator===  OutDataTypeStr=boolean  RndMeth=Simplest  InputSameDT=off
  z2 : Outport
  wires:
  Relational Operator1/1 -> Multiport Switch/1
  Constant2/1 -> Relational Operator1/2
  Memory1/1 -> Multiport Switch/2
  Integrator/1 -> Memory1/1
  Relational Operator/1 -> Integrator/2
  Constant1/1 -> Integrator/1
  Memory/1 -> Relational Operator1/1, Relational Operator/2
  stare_control2/1 -> Memory/1, Relational Operator/1
  Constant/1 -> Multiport Switch/3
  Multiport Switch/1 -> z2/1

== system proj_ish/extended/Control bariera3 ==
  stare_control3 : Inport
  Constant : Constant  Value=0
  Constant1 : Constant
  Constant2 : Constant
  Integrator : Integrator  ExternalReset=rising
  Memory : Memory  InitialCondition=1
  Memory1 : Memory  InitialCondition=1
  Multiport Switch : MultiPortSwitch  DataPortOrder=Specify indices  Inputs=2  DataPortIndices={0,1}  SaturateOnIntegerOverflow=off  InputSameDT=off
  Relational Operator : RelationalOperator  Operator=~=  OutDataTypeStr=boolean  RndMeth=Simplest  InputSameDT=off
  Relational Operator1 : RelationalOperator  Operator===  OutDataTypeStr=boolean  RndMeth=Simplest  InputSameDT=off
  z3 : Outport
  wires:
  Multiport Switch/1 -> z3/1
  Constant/1 -> Multiport Switch/3
  stare_control3/1 -> Relational Operator/1, Memory/1
  Memory/1 -> Relational Operator/2, Relational Operator1/1
  Constant1/1 -> Integrator/1
  Relational Operator/1 -> Integrator/2
  Integrator/1 -> Memory1/1
  Memory1/1 -> Multiport Switch/2
  Constant2/1 -> Relational Operator1/2
  Relational Operator1/1 -> Multiport Switch/1

== system proj_ish/extended/Control bariera4 ==
  stare_control4 : Inport
  Constant : Constant  Value=0
  Constant1 : Constant
  Constant2 : Constant
  Integrator : Integrator  ExternalReset=rising
  Memory : Memory  InitialCondition=1
  Memory1 : Memory  InitialCondition=1
  Multiport Switch : MultiPortSwitch  DataPortOrder=Specify indices  Inputs=2  DataPortIndices={0,1}  SaturateOnIntegerOverflow=off  InputSameDT=off
  Relational Operator : RelationalOperator  Operator=~=  OutDataTypeStr=boolean  RndMeth=Simplest  InputSameDT=off
  Relational Operator1 : RelationalOperator  Operator===  OutDataTypeStr=boolean  RndMeth=Simplest  InputSameDT=off
  z4 : Outport
  wires:
  Relational Operator1/1 -> Multiport Switch/1
  Constant2/1 -> Relational Operator1/2
  Memory1/1 -> Multiport Switch/2
  Integrator/1 -> Memory1/1
  Relational Operator/1 -> Integrator/2
  Constant1/1 -> Integrator/1
  Memory/1 -> Relational Operator1/1, Relational Operator/2
  stare_control4/1 -> Memory/1, Relational Operator/1
  Constant/1 -> Multiport Switch/3
  Multiport Switch/1 -> z4/1

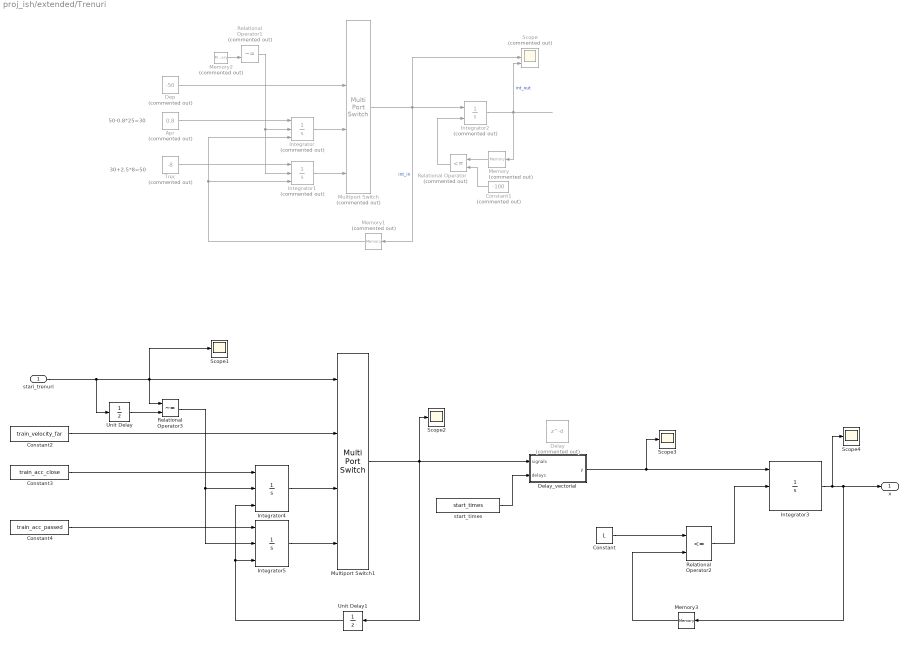
== system proj_ish/extended/Trenuri ==
  note: 30+2.5*8=50
  note: 50-0.8*25=30
  stari_trenuri : Inport
  Apr : Constant  Commented=on  Value=0.8
  Constant : Constant  Value=L
  Constant1 : Constant  Commented=on  Value=-100
  Constant2 : Constant  Value=train_velocity_far
  Constant3 : Constant  Value=train_acc_close
  Constant4 : Constant  Value=train_acc_passed
  Delay : Delay  Commented=on  DelayLengthSource=Input port
      settings: InputPortMap=u0,p1
  Delay_vectorial : MATLAB Function  TreatAsAtomicUnit=on
  Dep : Constant  Commented=on  Value=-50
  Integrator : Integrator  Commented=on  ExternalReset=rising  InitialConditionSource=external
  Integrator1 : Integrator  Commented=on  ExternalReset=rising  InitialConditionSource=external
  Integrator2 : Integrator  Commented=on  ExternalReset=rising  InitialCondition=4900
  Integrator3 : Integrator  ExternalReset=rising  InitialConditionSource=external
  Integrator4 : Integrator  ExternalReset=rising  InitialConditionSource=external  InitialCondition=50  LimitOutput=on  UpperSaturationLimit=60  LowerSaturationLimit=30
  Integrator5 : Integrator  ExternalReset=rising  InitialConditionSource=external  LimitOutput=on  UpperSaturationLimit=60  LowerSaturationLimit=30
  Memory : Memory  Commented=on
  Memory1 : Memory  Commented=on
  Memory2 : Memory  Commented=on  InitialCondition=1
  Memory3 : Memory
  Multiport Switch : MultiPortSwitch  Commented=on  SaturateOnIntegerOverflow=off  InputSameDT=off
  Multiport Switch1 : MultiPortSwitch  SaturateOnIntegerOverflow=off  InputSameDT=off
  Relational Operator : RelationalOperator  Commented=on  Operator=<=  OutDataTypeStr=boolean  RndMeth=Simplest  InputSameDT=off
  Relational Operator1 : RelationalOperator  Commented=on  Operator=~=  OutDataTypeStr=boolean  RndMeth=Simplest  InputSameDT=off
  Relational Operator2 : RelationalOperator  Operator=<=  OutDataTypeStr=boolean  RndMeth=Simplest  InputSameDT=off
  Relational Operator3 : RelationalOperator  Operator=~=  OutDataTypeStr=boolean  RndMeth=Simplest  InputSameDT=off
  Scope : Scope  Commented=on  NumInputPorts=3
  Scope{1..4} (4 alike) : Scope
  Trec : Constant  Commented=on  Value=-8
  Unit Delay : UnitDelay  InitialCondition=ones(1,trains)  SampleTime=-1  HasFrameUpgradeWarning=on
  Unit Delay1 : UnitDelay  InitialCondition=50  SampleTime=-1  HasFrameUpgradeWarning=on
  start_times : Constant  Value=start_times
  x : Outport
  wires:
  Dep/1 -> Multiport Switch/2
  ? -> Memory2/1, Scope/1, Multiport Switch/1, Relational Operator1/1
  Apr/1 -> Integrator/1
  Trec/1 -> Integrator1/1
  Integrator2/1 -> Scope/3, Memory/1  "int_out"
  Constant1/1 -> Relational Operator/2
  Memory/1 -> Relational Operator/1
  Relational Operator/1 -> Integrator2/2
  Multiport Switch/1 -> Scope/2, Memory1/1, Integrator2/1  "int_in"
  Integrator/1 -> Multiport Switch/3
  Integrator1/1 -> Multiport Switch/4
  Memory1/1 -> Integrator/3, Integrator1/3
  Memory2/1 -> Relational Operator1/2
  Relational Operator1/1 -> Integrator/2, Integrator1/2
  Multiport Switch1/1 -> Scope2/1, Unit Delay1/1, Delay_vectorial/1(signals)
  stari_trenuri/1 -> Multiport Switch1/1, Scope1/1, Relational Operator3/1, Unit Delay/1
  Integrator3/1 -> Memory3/1, x/1, Scope4/1
  Constant2/1 -> Multiport Switch1/2
  start_times/1 -> Delay_vectorial/2(delays)
  Integrator4/1 -> Multiport Switch1/3
  Integrator5/1 -> Multiport Switch1/4
  Delay_vectorial/1(y) -> Scope3/1, Integrator3/1
  Memory3/1 -> Relational Operator2/2
  Constant/1 -> Relational Operator2/1
  Relational Operator2/1 -> Integrator3/2
  Constant3/1 -> Integrator4/1
  Constant4/1 -> Integrator5/1
  Unit Delay/1 -> Relational Operator3/2
  Relational Operator3/1 -> Integrator5/2, Integrator4/2
  Unit Delay1/1 -> Integrator4/3, Integrator5/3

== system proj_ish/extended/Vehicle ==
  Throttle : Inport
  Brake : Inport  Port=2
  Engine : Subsystem
  PlotResults : Scope  NumInputPorts=3
  ShiftLogic : Stateflow chart  TreatAsAtomicUnit=on
  Transmission : Subsystem
  Vehicle : Subsystem  mask(vehicle model){Rfd=vehicledata(1), rload0=vehicledata(2), rload2=vehicledata(3), Rw=vehicledata(4), Iv=vehicledata(5), N20=vehicledata(6)/vehicledata(4)*vehicledata(1)}
      mask prompts: Rfd "final drive ratio"; rload0 "drag friction at wheels"; rload2 "aerodynamic drag"; Rw "wheel radius"; Iv "vehicle inertia"; N20 "initial transmission output speed"
      mask help: vehicle dynamics: torque input from trans., outputs are input speed (transmission output) and vehicle speed
      mask Display: image('$imagefile') % use "Edit Image" on toolstrip to change.
  VehicleSpeed : Outport
  EngineRPM : Outport  Port=2
  wires:
  Engine/1(Ne) -> Transmission/1(Ne), EngineRPM/1, PlotResults/2  "EngineRPM"
  Vehicle/2(TransmissionRPM) -> Transmission/3(Nout)  "TransmissionRPM"
  Transmission/1(Ti) -> Engine/1(Ti)  "ImpellerTorque"
  Brake/1 -> Vehicle/2(BrakeTorque)  "Brake"
  Vehicle/1(VehicleSpeed) -> ShiftLogic/2(VehicleSpeed), VehicleSpeed/1, PlotResults/3  "VehicleSpeed"
  Transmission/2(Tout) -> Vehicle/1(OutputTorque)  "OutputTorque"
  ShiftLogic/1(Gear) -> Transmission/2(Gear)
  Throttle/1 -> Engine/2(Throttle), PlotResults/1, ShiftLogic/1(Throttle)  "Throttle"

== system proj_ish/Cars/Transmission/TorqueConverter ==
  note: Torque Converter
  Ne : Inport
  Nin : Inport  Port=2
  FactorK : Lookup_n-D  NumberOfTableDimensions=1  BreakpointsForDimension1=speedratio  Table=Kfactor  SaturateOnIntegerOverflow=on
  Impeller : Fcn  Expr=u^2
  Quotient : Product  Inputs=*/  InputSameDT=on  SaturateOnIntegerOverflow=on  OutDataTypeStr=Inherit: Same as first input
  SpeedRatio : Product  Inputs=*/  InputSameDT=on  SaturateOnIntegerOverflow=on  OutDataTypeStr=Inherit: Same as first input
  TorqueRatio : Lookup_n-D  NumberOfTableDimensions=1  BreakpointsForDimension1=speedratio  Table=Torkratio  SaturateOnIntegerOverflow=on
  Turbine : Product  InputSameDT=on  SaturateOnIntegerOverflow=on  OutDataTypeStr=Inherit: Same as first input
  Ti : Outport  VectorParamsAs1DForOutWhenUnconnected=off
  Tt : Outport  Port=2  VectorParamsAs1DForOutWhenUnconnected=off
  wires:
  TorqueRatio/1 -> Turbine/2
  Quotient/1 -> Impeller/1
  FactorK/1 -> Quotient/2
  SpeedRatio/1 -> TorqueRatio/1, FactorK/1
  Impeller/1 -> Turbine/1, Ti/1
  Turbine/1 -> Tt/1
  Ne/1 -> SpeedRatio/2, Quotient/1
  Nin/1 -> SpeedRatio/1

== system proj_ish/Cars/Transmission/TransmissionRatio ==
  note: Transmission Gear Ratio
  Tin : Inport  Unit=ft*lbf@torque
  Gear : Inport  Port=2  Unit=1
  Nout : Inport  Port=3  Unit=rpm
  Product : Product  InputSameDT=on  SaturateOnIntegerOverflow=on  OutDataTypeStr=Inherit: Same as first input
  Product1 : Product  InputSameDT=on  SaturateOnIntegerOverflow=on  OutDataTypeStr=Inherit: Same as first input
  Table : Lookup_n-D  NumberOfTableDimensions=1  BreakpointsForDimension1=[1 2 3 4]  Table=[2.393 1.450 1.000 0.677]  ExtrapMethod=Clip  OutDataTypeStr=double  SaturateOnIntegerOverflow=on  LockScale=on
  Tout : Outport  Unit=ft*lbf@torque  VectorParamsAs1DForOutWhenUnconnected=off
  Nin : Outport  Port=2  Unit=rpm  VectorParamsAs1DForOutWhenUnconnected=off
  wires:
  Table/1 -> Product1/1, Product/2
  Nout/1 -> Product1/2
  Product1/1 -> Nin/1
  Product/1 -> Tout/1
  Tin/1 -> Product/1
  Gear/1 -> Table/1

== system proj_ish/Cars/Vehicle/WheelSpeedToLinearSpeed ==
  WS : Inport  Unit=rpm
  ToLinearSpeed : Gain  Gain=2*pi*Rw  SaturateOnIntegerOverflow=on  OutDataTypeStr=Inherit: Same as input  ParamDataTypeStr=Inherit: Same as input
  LS : Outport  Unit=ft/min  VectorParamsAs1DForOutWhenUnconnected=off
  wires:
  ToLinearSpeed/1 -> LS/1
  WS/1 -> ToLinearSpeed/1

== system proj_ish/extended/Vehicle/Engine ==
  note: Engine
  Ti : Inport  Unit=ft*lbf@torque
  Throttle : Inport  Port=2  Unit=%
  EnginePlusImpellerInertia : Gain  Gain=1/Iei  SaturateOnIntegerOverflow=on  OutDataTypeStr=Inherit: Same as input  ParamDataTypeStr=Inherit: Same as input
  EngineTorque : Lookup_n-D  BreakpointsForDimension1=thvec  BreakpointsForDimension2=nevec  Table=emap
      settings: InputPortMap=u0,u1
  Integrator : Integrator  InitialCondition=1000  LimitOutput=on  UpperSaturationLimit=6000  LowerSaturationLimit=600  ZeroCross=off
  Sum : Sum  Inputs=-+  InputSameDT=on  SaturateOnIntegerOverflow=on  OutDataTypeStr=Inherit: Same as first input
  Ne : Outport  Unit=rpm  VectorParamsAs1DForOutWhenUnconnected=off
  wires:
  Ti/1 -> Sum/1
  Throttle/1 -> EngineTorque/1
  Integrator/1 -> EngineTorque/2, Ne/1
  Sum/1 -> EnginePlusImpellerInertia/1
  EnginePlusImpellerInertia/1 -> Integrator/1
  EngineTorque/1 -> Sum/2

== system proj_ish/extended/Vehicle/ShiftLogic/ComputeThreshold ==
  note: Threshold Calculation
  Gear : Inport
  Throttle : Inport  Port=2
  f : TriggerPort  TriggerType=function-call  VariantControl=(inherit)
      settings: CopyFcn=Stateflow.SLINSF.SimulinkMan.removeBlockPreDeleteFcn  PreDeleteFcn=Stateflow.SLINSF.SimulinkMan.unsafePredeleteFcn
  InterpDown : Lookup_n-D  BreakpointsForDimension1=downth  BreakpointsForDimension2=[1:4]  Table=downtab  OutDataTypeStr=double  InputSameDT=off  LockScale=on
      settings: InputPortMap=u0,u1
  InterpUp : Lookup_n-D  BreakpointsForDimension1=upth  BreakpointsForDimension2=[1:4]  Table=uptab  OutDataTypeStr=double  InputSameDT=off  LockScale=on
      settings: InputPortMap=u0,u1
  down_th : Outport  InitialOutput=0  VectorParamsAs1DForOutWhenUnconnected=off
  up_th : Outport  Port=2  InitialOutput=0  VectorParamsAs1DForOutWhenUnconnected=off
  wires:
  InterpUp/1 -> up_th/1
  InterpDown/1 -> down_th/1
  Throttle/1 -> InterpDown/1, InterpUp/1
  Gear/1 -> InterpDown/2, InterpUp/2

== system proj_ish/extended/Vehicle/Transmission ==
  note: Transmission
  Ne : Inport  Unit=rpm
  Gear : Inport  Port=2  Unit=1
  Nout : Inport  Port=3  Unit=rpm
  TorqueConverter : Subsystem  mask(torque converter){speedratio=converter_data(:,1), Kfactor=converter_data(:,2), Torkratio=converter_data(:,3)}
      mask prompts: speedratio "speed ratio"; Kfactor "K factor"; Torkratio "torque ratio"
      mask help: torque converter
      mask Help: Torque converter input and output torques are computed as a function of the input and output speeds
      mask Display: plot([cos([90:10:450]*pi/180),.63*cos([90:10:450]*pi/180),.63*cos([90:10:240]*pi/180),cos([240:10:300]*pi/180),.63*cos([300]*pi/180)],[sin([90:10:450]*pi/180),.63*sin([90:10:450]*pi/180)+.1,.63*sin([90:10:240]*pi/180)+.1,sin([240:10:300]*pi/180),.63*sin([300]*pi/180)+.1])
  TransmissionRatio : Subsystem
  Ti : Outport  Unit=ft*lbf@torque  VectorParamsAs1DForOutWhenUnconnected=off
  Tout : Outport  Port=2  Unit=ft*lbf@torque  VectorParamsAs1DForOutWhenUnconnected=off
  wires:
  TransmissionRatio/1(Tout) -> Tout/1
  TorqueConverter/1(Ti) -> Ti/1
  Nout/1 -> TransmissionRatio/3(Nout)
  Gear/1 -> TransmissionRatio/2(Gear)
  Ne/1 -> TorqueConverter/1(Ne)
  TransmissionRatio/2(Nin) -> TorqueConverter/2(Nin)
  TorqueConverter/2(Tt) -> TransmissionRatio/1(Tin)  "TurbineTorque"

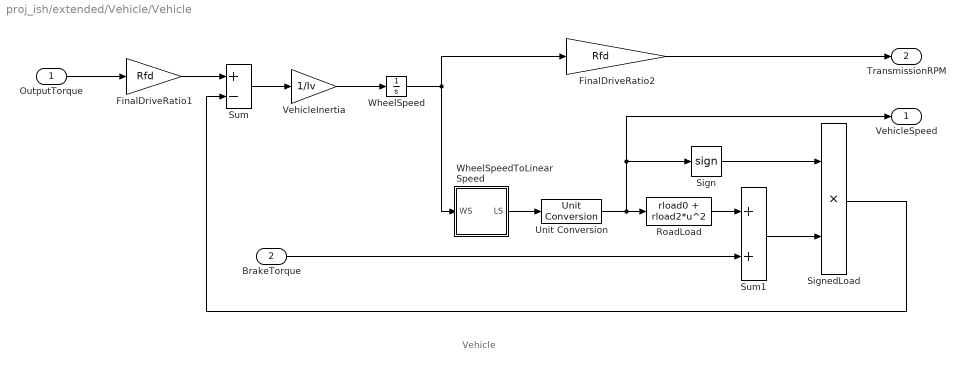
== system proj_ish/extended/Vehicle/Vehicle ==
  note: Vehicle
  OutputTorque : Inport  Unit=ft*lbf@torque
  BrakeTorque : Inport  Port=2  Unit=ft*lbf@torque
  FinalDriveRatio1 : Gain  Gain=Rfd  SaturateOnIntegerOverflow=on  OutDataTypeStr=Inherit: Same as input  ParamDataTypeStr=Inherit: Same as input
  FinalDriveRatio2 : Gain  Gain=Rfd  SaturateOnIntegerOverflow=on  OutDataTypeStr=Inherit: Same as input  ParamDataTypeStr=Inherit: Same as input
  RoadLoad : Fcn  Expr=rload0 + rload2*u^2
  Sign : Signum
  SignedLoad : Product  InputSameDT=on  SaturateOnIntegerOverflow=on  OutDataTypeStr=Inherit: Same as first input
  Sum : Sum  Inputs=+-  InputSameDT=on  SaturateOnIntegerOverflow=on  OutDataTypeStr=Inherit: Same as first input
  Sum1 : Sum  InputSameDT=on  SaturateOnIntegerOverflow=on  OutDataTypeStr=Inherit: Same as first input
  Unit Conversion : UnitConversion
  VehicleInertia : Gain  Gain=1/Iv  SaturateOnIntegerOverflow=on  OutDataTypeStr=Inherit: Same as input  ParamDataTypeStr=Inherit: Same as input
  WheelSpeed : Integrator  InitialCondition=N20/Rfd  ZeroCross=off
  WheelSpeedToLinearSpeed : Subsystem
  VehicleSpeed : Outport  Unit=mph  VectorParamsAs1DForOutWhenUnconnected=off
  TransmissionRPM : Outport  Port=2  Unit=rpm  VectorParamsAs1DForOutWhenUnconnected=off
  wires:
  FinalDriveRatio2/1 -> TransmissionRPM/1
  BrakeTorque/1 -> Sum1/2
  Sum1/1 -> SignedLoad/2
  RoadLoad/1 -> Sum1/1
  Sign/1 -> SignedLoad/1
  SignedLoad/1 -> Sum/2
  OutputTorque/1 -> FinalDriveRatio1/1
  VehicleInertia/1 -> WheelSpeed/1
  Sum/1 -> VehicleInertia/1
  Unit Conversion/1 -> VehicleSpeed/1, Sign/1, RoadLoad/1
  WheelSpeed/1 -> WheelSpeedToLinearSpeed/1(WS), FinalDriveRatio2/1
  FinalDriveRatio1/1 -> Sum/1
  WheelSpeedToLinearSpeed/1(LS) -> Unit Conversion/1

== system proj_ish/extended/Vehicle/Transmission/TorqueConverter ==
  note: Torque Converter
  Ne : Inport
  Nin : Inport  Port=2
  FactorK : Lookup_n-D  NumberOfTableDimensions=1  BreakpointsForDimension1=speedratio  Table=Kfactor  SaturateOnIntegerOverflow=on
  Impeller : Fcn  Expr=u^2
  Quotient : Product  Inputs=*/  InputSameDT=on  SaturateOnIntegerOverflow=on  OutDataTypeStr=Inherit: Same as first input
  SpeedRatio : Product  Inputs=*/  InputSameDT=on  SaturateOnIntegerOverflow=on  OutDataTypeStr=Inherit: Same as first input
  TorqueRatio : Lookup_n-D  NumberOfTableDimensions=1  BreakpointsForDimension1=speedratio  Table=Torkratio  SaturateOnIntegerOverflow=on
  Turbine : Product  InputSameDT=on  SaturateOnIntegerOverflow=on  OutDataTypeStr=Inherit: Same as first input
  Ti : Outport  VectorParamsAs1DForOutWhenUnconnected=off
  Tt : Outport  Port=2  VectorParamsAs1DForOutWhenUnconnected=off
  wires:
  TorqueRatio/1 -> Turbine/2
  Quotient/1 -> Impeller/1
  FactorK/1 -> Quotient/2
  SpeedRatio/1 -> TorqueRatio/1, FactorK/1
  Impeller/1 -> Turbine/1, Ti/1
  Turbine/1 -> Tt/1
  Ne/1 -> SpeedRatio/2, Quotient/1
  Nin/1 -> SpeedRatio/1

== system proj_ish/extended/Vehicle/Transmission/TransmissionRatio ==
  note: Transmission Gear Ratio
  Tin : Inport  Unit=ft*lbf@torque
  Gear : Inport  Port=2  Unit=1
  Nout : Inport  Port=3  Unit=rpm
  Product : Product  InputSameDT=on  SaturateOnIntegerOverflow=on  OutDataTypeStr=Inherit: Same as first input
  Product1 : Product  InputSameDT=on  SaturateOnIntegerOverflow=on  OutDataTypeStr=Inherit: Same as first input
  Table : Lookup_n-D  NumberOfTableDimensions=1  BreakpointsForDimension1=[1 2 3 4]  Table=[2.393 1.450 1.000 0.677]  ExtrapMethod=Clip  OutDataTypeStr=double  SaturateOnIntegerOverflow=on  LockScale=on
  Tout : Outport  Unit=ft*lbf@torque  VectorParamsAs1DForOutWhenUnconnected=off
  Nin : Outport  Port=2  Unit=rpm  VectorParamsAs1DForOutWhenUnconnected=off
  wires:
  Table/1 -> Product1/1, Product/2
  Nout/1 -> Product1/2
  Product1/1 -> Nin/1
  Product/1 -> Tout/1
  Tin/1 -> Product/1
  Gear/1 -> Table/1
